simulink model "TL_model_4"  (R2015b)
settings: Solver=VariableStepAuto  StartTime=0.0  StopTime=50  RelTol=1e-3
settings Model: Creator=loicgelle  LastModifiedBy=loicgelle

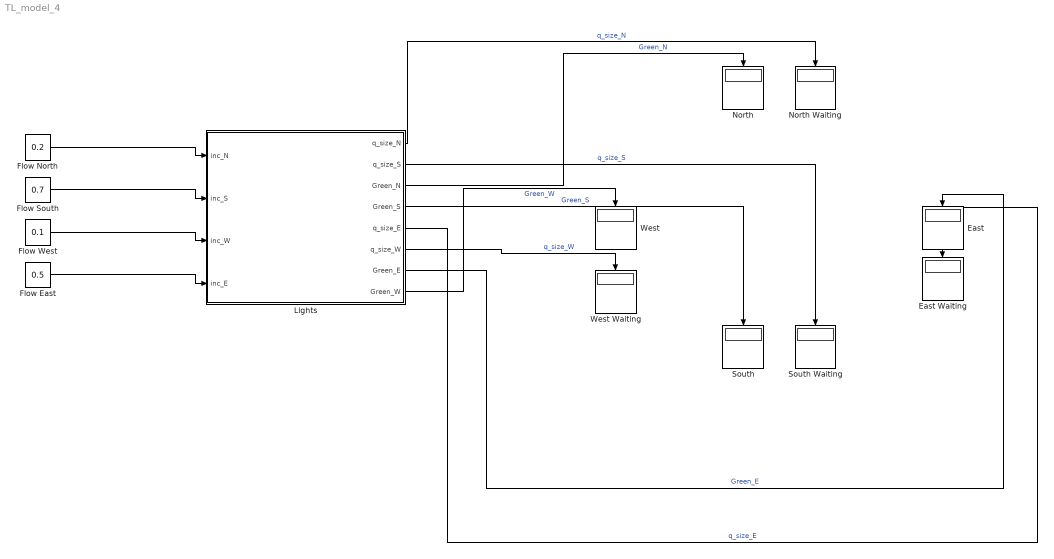
== system TL_model_4 ==
  " East" : Display
  " East Waiting" : Display
  " North" : Display
  " North Waiting" : Display
  " South" : Display
  " South Waiting" : Display
  " West" : Display
  " West Waiting" : Display
  Flow East : Constant  Value=0.5
  Flow North : Constant  Value=0.2
  Flow South : Constant  Value=0.7
  Flow West : Constant  Value=0.1
  Lights : Stateflow chart  TreatAsAtomicUnit=on  VariantControl=Variant1
  wires:
  Lights/3(Green_N) -> " North"/1  "Green_N"
  Lights/4(Green_S) -> " South"/1  "Green_S"
  Flow North/1 -> Lights/1(inc_N)
  Flow South/1 -> Lights/2(inc_S)
  Lights/2(q_size_S) -> " South Waiting"/1  "q_size_S"
  Lights/1(q_size_N) -> " North Waiting"/1  "q_size_N"
  Flow West/1 -> Lights/3(inc_W)
  Flow East/1 -> Lights/4(inc_E)
  Lights/7(Green_E) -> " East"/1  "Green_E"
  Lights/8(Green_W) -> " West"/1  "Green_W"
  Lights/6(q_size_W) -> " West Waiting"/1  "q_size_W"
  Lights/5(q_size_E) -> " East Waiting"/1  "q_size_E"

== stateflow chart TL_model_4/Lights ==
  settings: updateMethod=CONTINUOUS
  state LightsController [parallel]
    settings: executionOrder=1
    state GreenS
      entry:
      t = 0;
      Green_S = 1;
      during:
      t_dot = 1;
      exit:
      Green_S = 0;
    state Green_E
      entry:
      t = 0;
      Green_E = 1;
      during:
      t_dot = 1;
      exit:
      Green_E = 0;
    state GreenN
      entry:
      t = 0;
      Green_N = 1;
      during:
      t_dot = 1;
      exit:
      Green_N = 0;
    state GreenW
      entry:
      t = 0;
      Green_W = 1;
      during:
      t_dot = 1;
      exit:
      Green_W = 0;
    state Clear
      entry:
      Green_N = 0;
      Green_S = 0;
      Green_E = 0;
      Green_W = 0;
    GreenS -> Clear [order 1] : [t >= t_S]
    Green_E -> GreenS [order 2] : [t >= t_E]
    GreenN -> Green_E [order 2] : [t >= t_N]
    GreenW -> GreenN [order 1] : [t >= t_W]
    Clear -> GreenW [order 2] : after(1, sec)
        | [q_size_N + q_size_S + q_size_E + q_size_W > 0]
        | {computeTimes()}
    GreenN -> Green_E [order 1] : [q_size_N <= 0]
    Green_E -> GreenS [order 1] : [q_size_E <= 0]
    GreenW -> GreenN [order 2] : [q_size_W <= 0]
    GreenS -> Clear [order 2] : [q_size_S <= 0]
    Clear -> Clear [order 1] : after(1, sec)
        | [q_size_N + q_size_S + q_size_W + q_size_E <= 0]
    (default) -> Clear
  state Queue_Handler_N [parallel]
    settings: executionOrder=2
    state Red
      during:
      q_size_N_dot = inc_N;
    state Green
      during:
      q_size_N_dot = inc_N - out;
    Queue_Handler_N.Green -> Queue_Handler_N.Red : [Green_N == 0]
    Queue_Handler_N.Red -> Queue_Handler_N.Green : [Green_N == 1]
    (default) -> Queue_Handler_N.Red
  state Queue_Handler_S [parallel]
    settings: executionOrder=3
    state Red
      during:
      q_size_S_dot = inc_S;
    state Green
      during:
      q_size_S_dot = inc_S - out;
    Queue_Handler_S.Green -> Queue_Handler_S.Red : [Green_S == 0]
    Queue_Handler_S.Red -> Queue_Handler_S.Green : [Green_S == 1]
    (default) -> Queue_Handler_S.Red
  state Queue_Handler_E [parallel]
    settings: executionOrder=4
    state Red
      during:
      q_size_E_dot = inc_E;
    state Green
      during:
      q_size_E_dot = inc_E - out;
    Queue_Handler_E.Green -> Queue_Handler_E.Red : [Green_E == 0]
    Queue_Handler_E.Red -> Queue_Handler_E.Green : [Green_E == 1]
    (default) -> Queue_Handler_E.Red
  state Queue_Handler_S1 [parallel]
    settings: executionOrder=5
    state Red
      during:
      q_size_W_dot = inc_W;
    state Green
      during:
      q_size_W_dot = inc_W - out;
    Queue_Handler_S1.Green -> Queue_Handler_S1.Red : [Green_W == 0]
    Queue_Handler_S1.Red -> Queue_Handler_S1.Green : [Green_W == 1]
    (default) -> Queue_Handler_S1.Red
  data: q_size_N output =0; q_size_S output =0; t_N local =0; t_S local =0; cycle_duration constant double =10; Green_N output; Green_S output; data local; inc_N input; inc_S input; out constant double =2; t local =0; t_E local =0; q_size_E output =0; q_size_W output =0; inc_W input; inc_E input; Green_E output; Green_W output; t_W local =0
  data q_size_N settings: updateMethod=SF_CONTINUOUS_TIME_DATA
  data q_size_S settings: updateMethod=SF_CONTINUOUS_TIME_DATA
  data t settings: updateMethod=SF_CONTINUOUS_TIME_DATA
  data q_size_E settings: updateMethod=SF_CONTINUOUS_TIME_DATA
  data q_size_W settings: updateMethod=SF_CONTINUOUS_TIME_DATA
  function computeTimes:
    | function computeTimes
    | 
    | Q = q_size_E + q_size_N + q_size_W + q_size_S;
    | t_N = q_size_N * cycle_duration / (4*Q);
    | t_S = q_size_S * cycle_duration / (4*Q);
    | t_W = q_size_W * cycle_duration / (4*Q);
    | t_E = q_size_E * cycle_duration / (4*Q);
